simulink model "MDL_example001"  (Simulink 9.1)
settings: Solver=FixedStepDiscrete  StartTime=0.0  StopTime=N  FixedStep=Ts  RelTol=1e-3
values from neighbouring files (symbols this model uses):
  Ts = 0.1    [Cal_input.m]
settings Model: Creator=80741  LastModifiedBy=80741
settings DataIOCC: LimitDataPoints=on  SignalLoggingSaveFormat=ModelDataLogs
settings OptimizationCC: InitFltsAndDblsToZero=on
settings DebuggingCC: SaveWithParameterizedLinksMsg=none  SignalResolutionControl=TryResolveAllWithWarning  SolverPrmCheckMsg=warning  MultiTaskDSMMsg=warning  MultiTaskCondExecSysMsg=none  FcnCallInpInsideContextMsg=warning
settings GRTTargetCC: TargetFcnLib=ansi_tfl_tmw.mat

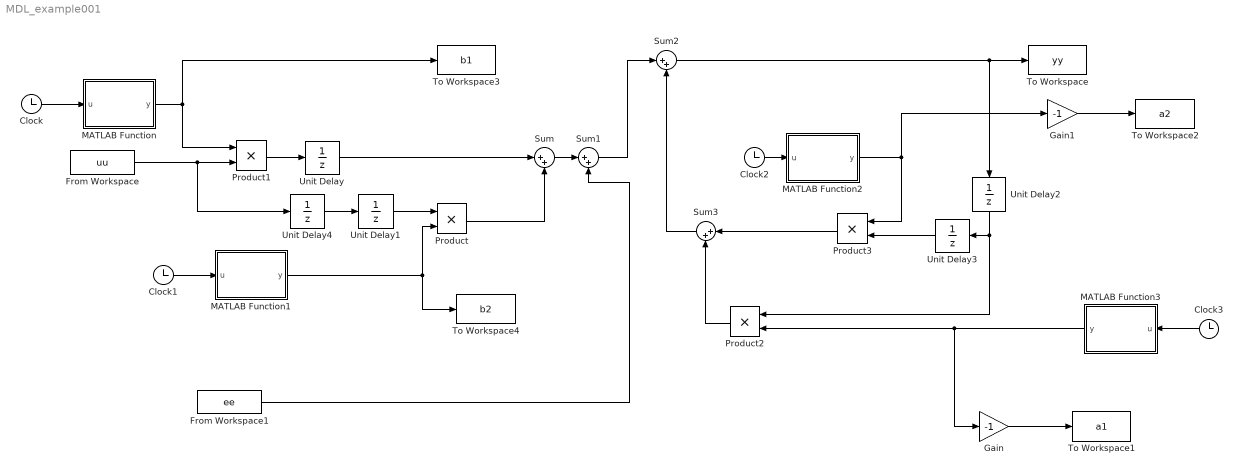
== system MDL_example001 ==
  Clock{,1..3} (4 alike) : Clock
  From Workspace : FromWorkspace  VariableName=uu  SampleTime=Ts
  From Workspace1 : FromWorkspace  VariableName=ee  SampleTime=Ts
  Gain : Gain  Gain=-1
  Gain1 : Gain  Gain=-1
  MATLAB Function : MATLAB Function  TreatAsAtomicUnit=on
  MATLAB Function1 : MATLAB Function  TreatAsAtomicUnit=on
  MATLAB Function2 : MATLAB Function  TreatAsAtomicUnit=on
  MATLAB Function3 : MATLAB Function  TreatAsAtomicUnit=on
  Product{,1..3} (4 alike) : Product  RndMeth=Zero
  Sum{,1..3} (4 alike) : Sum  Inputs=|++
  To Workspace : ToWorkspace  VariableName=yy  SampleTime=Ts
  To Workspace1 : ToWorkspace  VariableName=a1  SampleTime=Ts
  To Workspace2 : ToWorkspace  VariableName=a2  SampleTime=Ts
  To Workspace3 : ToWorkspace  VariableName=b1  SampleTime=Ts
  To Workspace4 : ToWorkspace  VariableName=b2  SampleTime=Ts
  Unit Delay{,1..4} (5 alike) : UnitDelay  SampleTime=Ts
  wires:
  Unit Delay/1 -> Sum/1
  Sum/1 -> Sum1/1
  From Workspace1/1 -> Sum1/2
  Sum1/1 -> Sum2/1
  Sum2/1 -> To Workspace/1, Unit Delay2/1
  Unit Delay2/1 -> Unit Delay3/1, Product2/1
  Unit Delay3/1 -> Product3/2
  Sum3/1 -> Sum2/2
  Product3/1 -> Sum3/1
  Product/1 -> Sum/2
  MATLAB Function1/1(y) -> Product/2, To Workspace4/1
  Product1/1 -> Unit Delay/1
  MATLAB Function/1(y) -> To Workspace3/1, Product1/1
  Product2/1 -> Sum3/2
  MATLAB Function3/1(y) -> Product2/2, Gain/1
  MATLAB Function2/1(y) -> Product3/1, Gain1/1
  Unit Delay4/1 -> Unit Delay1/1
  Unit Delay1/1 -> Product/1
  Gain/1 -> To Workspace1/1
  Gain1/1 -> To Workspace2/1
  From Workspace/1 -> Product1/2, Unit Delay4/1
  Clock/1 -> MATLAB Function/1(u)
  Clock1/1 -> MATLAB Function1/1(u)
  Clock2/1 -> MATLAB Function2/1(u)
  Clock3/1 -> MATLAB Function3/1(u)

== matlab function MATLAB Function1 ==
  data: u input double; y output double
function y = fcn(u)
if(u>5)
    y=0.06182;
elseif(u>2)
    y=0.09272;
else
    y=0.1236;
end

== matlab function MATLAB Function ==
  data: u input double; y output double
function y = fcn(u)
if(u>5)
    y=-0.06485;
elseif(u>2)
    y=-0.09728;
else
    y=-0.1297;
end

== matlab function MATLAB Function2 ==
  data: u input double; y output double
function y = fcn(u)
y=-0.9427;
end

== matlab function MATLAB Function3 ==
  data: u input double; y output double
function y = fcn(u)
y=1.961;
end
